simulink model "Transmitter"  (R2017b)
settings: Solver=FixedStepDiscrete  StartTime=0.0  StopTime=10  RelTol=1e-3
InitFcn:
  | numHeaderBits = 16;
  | %numPreambleBits = 250;
  | AGCBarkerSymbols = 160+28;
  | EQTrainingSymbols = 250;
  | CRCGeneratorLag = 34; % CRCLen + 2
  | 
  | %% AGC Preamble
  | B13bipolar = [0 0 0 0 0 2 2 0 0 2 0 2];
  | rep = [B13bipolar, B13bipolar(1:4)];
  | AGCBarker = repmat(rep,1,10);
  | % Second preamble part
  | B11bipolar = [0 0 0 2 2 2 0 2  2 0 2];
  | TimingBarker = [B11bipolar,B11bipolar,B11bipolar,B11bipolar(1:6)];
  | PreambleBarkersInts = [AGCBarker, TimingBarker];
  | % Convert integer into their bit representation
  | PreambleBarkersBits = zeros(1,length(PreambleBarkersInts)*2);
  | PreambleBarkersBits(1:2:end) = (PreambleBarkersInts==2);
  | 
  | % Constants
  | % First preamble part
  | B13bipolar = [0 0 0 0 0 2 2 0 0 2 0 2];
  | rep = [B13bipolar, B13bipolar(1:4)];
  | AGCBarker = repmat(rep,1,10);
  | % Second preamble part
  | B11bipolar = [0 0 0 2 2 2 0 2  2 0 2];
  | TimingBarker = [B11bipolar,B11bipolar,B11bipolar(1:6)];
  | PreambleBarkersInts = [AGCBarker, TimingBarker];
  | % Convert integer into their bit representation
  | PreambleBarkersBits = false(1,length(PreambleBarkersInts)*2);
  | PreambleBarkersBits(1:2:end) = logical(PreambleBarkersInts==2);
  | pLen = uint16(length(PreambleBarkersBits));
libraries: dspsigops x2, RxTxFixedPointLibrary x1
settings Model: DataTypeOverride=Off  Creator=tcollins  LastModifiedBy=tcollins
settings DataIOCC: SaveOutput=off  SaveTime=off
settings OptimizationCC: BlockReduction=off  ConditionallyExecuteInputs=off  DefaultParameterBehavior=Inlined
settings DebuggingCC: AlgebraicLoopMsg=error  SingleTaskRateTransMsg=error  ParameterPrecisionLossMsg=none
settings HardwareCC: ProdBitPerPointer=32  ProdBitPerSizeT=32  ProdBitPerPtrDiffT=32  ProdLargestAtomicFloat=None  ProdIntDivRoundTo=Undefined  ProdEndianess=Unspecified  ProdWordSize=32  ProdHWDeviceType=ASIC/FPGA->ASIC/FPGA  ProdEqTarget=off
settings CodeAppCC: StateflowObjectComments=on
settings SimscapeCC: SimscapeNormalizeSystem=off

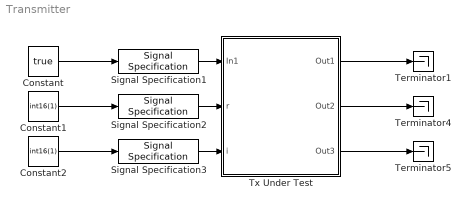
== system Transmitter ==
  Constant : Constant  Value=true  SampleTime=-1
  Constant1 : Constant  Value=int16(1)  SampleTime=-1
  Constant2 : Constant  Value=int16(1)  SampleTime=-1
  Signal Specification1 : SignalSpecification  OutDataTypeStr=boolean  SampleTime=1e-6
  Signal Specification2 : SignalSpecification  OutDataTypeStr=int16  SampleTime=1e-6
  Signal Specification3 : SignalSpecification  OutDataTypeStr=int16  SampleTime=1e-6
  Terminator1 : Terminator
  Terminator4 : Terminator
  Terminator5 : Terminator
  Tx Under Test : Subsystem  TreatAsAtomicUnit=on
      mask Display:
      | if ispc
      |     d = '\';
      | else
      |     d = '/';
      | end
      | model_path = get_param(bdroot, 'FileName');
      | %info = Simulink.MDLInfo(bdroot)
      | c = strsplit(model_path,d); c = c(1:end-2);c = strjoin(c,d)
      | logo = [c,d,'ADI_logo.svg'];
      | %disp(logo);
      | image(logo);
  wires:
  Constant/1 -> Signal Specification1/1
  Tx Under Test/1(Out1) -> Terminator1/1
  Tx Under Test/2(Out2) -> Terminator4/1
  Tx Under Test/3(Out3) -> Terminator5/1
  Signal Specification1/1 -> Tx Under Test/1(In1)
  Constant1/1 -> Signal Specification2/1
  Signal Specification2/1 -> Tx Under Test/2("r ")
  Constant2/1 -> Signal Specification3/1
  Signal Specification3/1 -> Tx Under Test/3(i)

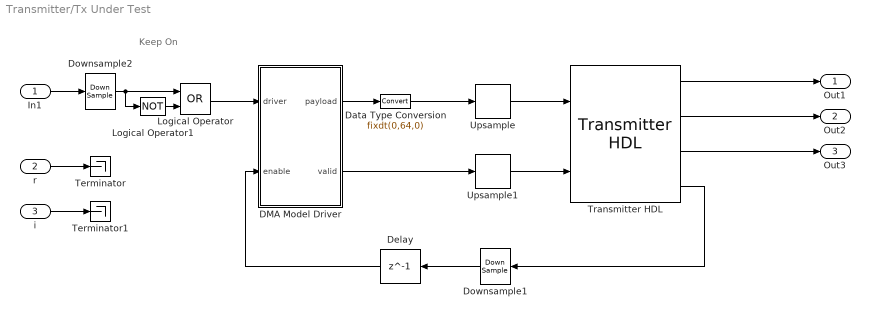
== system Transmitter/Tx Under Test ==
  note: Keep On
  In1 : Inport
  "r " : Inport  Port=2
  i : Inport  Port=3
  DMA Model Driver : MATLAB Function  TreatAsAtomicUnit=on
  Data Type Conversion : DataTypeConversion  OutDataTypeStr=fixdt(0,64,0)
  Delay : Delay  DelayLength=1
  Downsample1 : DownSample  N=4  RateOptions=Allow multirate processing
  Downsample2 : DownSample  N=4  RateOptions=Allow multirate processing
  Logical Operator : Logic  Operator=OR  AllPortsSameDT=off  OutDataTypeStr=boolean
  Logical Operator1 : Logic  Operator=NOT  AllPortsSameDT=off  OutDataTypeStr=boolean
  Terminator : Terminator
  Terminator1 : Terminator
  Transmitter HDL : RxTxFixedPointLibrary/Transmitter HDL  SystemSampleTime=-1
  Upsample : dspsigops/Upsample  N=4  phase=0  RateOptions=Allow multirate processing  ic=0  mode=Unused parameter value
  Upsample1 : dspsigops/Upsample  N=4  phase=0  RateOptions=Allow multirate processing  ic=0  mode=Unused parameter value
  Out1 : Outport
  Out2 : Outport  Port=2
  Out3 : Outport  Port=3
  wires:
  Transmitter HDL/4 -> Downsample1/1
  Transmitter HDL/2 -> Out2/1
  Transmitter HDL/1 -> Out1/1
  Transmitter HDL/3 -> Out3/1
  DMA Model Driver/1(payload) -> Data Type Conversion/1
  Delay/1 -> DMA Model Driver/2(enable)
  In1/1 -> Downsample2/1
  Data Type Conversion/1 -> Upsample/1
  DMA Model Driver/2(valid) -> Upsample1/1
  "r "/1 -> Terminator/1
  i/1 -> Terminator1/1
  Upsample/1 -> Transmitter HDL/1
  Upsample1/1 -> Transmitter HDL/2
  Downsample1/1 -> Delay/1
  Logical Operator/1 -> DMA Model Driver/1(driver)
  Logical Operator1/1 -> Logical Operator/2
  Downsample2/1 -> Logical Operator/1, Logical Operator1/1

== matlab function Transmitter/Tx Under Test/DMA Model Driver ==
  data: driver input; payload output; valid output boolean; enable input
function [payload,valid] = fcn(driver, enable)
%#codegen

persistent indx mode

pSize = fi(200,0,64,0); % Size in bytes (Must be multiple of 32 bits) cannot exceed uint16 max
mask = uint16(sum(2.^(0:15)));

if isempty(indx)
    indx = pSize;
    mode = int8(0);
end

% % Randomly dont transmit new data
% if enable && mode == 0
%    enable = randn>1; 
% end

if enable && driver
    valid = true;
    switch mode
        case int8(0) % Fresh packet start
%             disp('New Packet Start');
            payload = fi(pSize,0,64,0);%Upper bits
            mode = int8(1);
            indx = fi(0,0,64,0);
        otherwise%case 2
            indx = fi(indx + fi(8,0,64,0),0,64,0);
            %payload = uint32(sum(2.^[0 2 4 6 8 10 12 14 ]));
            if indx == fi(8,0,64,0)
                payload = fi(0,0,64,0);
            elseif indx == pSize
                payload = fi(uint64(18446744073709551615),0,64,0); % All ones
            else
                payload = fi(uint64(12297829382473034410),0,64,0);%sum(2.^[0:2:14])); % Alternating ones and zeros
            end
            
            if indx == pSize % reached end of frame
                mode = int8(0);
            end
    end
else
    valid = false;
    payload = fi(0,0,64,0);
end
